simulink model "regs_12B_with_contracts_All_SLDV"  (R2017b)
settings: Solver=FixedStepDiscrete  StartTime=0.0  StopTime=10.0  FixedStep=0.200000  RelTol=1e-3  EnableMultiTasking=on
model workspace (MAT data in the model file):
  ContractValidatorBlocksMap = containers.Map
  ContractValidatorBlocksMap.serialization.keys = {'regs_12B_with_contracts/regs_12B_RegulatorSpec/validator', 'regs_12B_with_contracts_All/regs_12B_RegulatorSpec/validator'}
  ContractValidatorBlocksMap.serialization.values{1}.block = 'regs_12B_with_contracts/regs_12B_RegulatorSpec/validator'
  ContractValidatorBlocksMap.serialization.values{1}.assumePorts = 0
  ContractValidatorBlocksMap.serialization.values{1}.guaranteePorts = 10
  ContractValidatorBlocksMap.serialization.values{1}.modeBlocksPorts = 0
  ContractValidatorBlocksMap.serialization.values{1}.portHandles.Inport = [5912.00012207 5913.00012207 5914.00012207 5915.00012207 5916.00012207 5917.00012207 5918.00012207 5919.00012207 5920.00012207 5921.00012207]
  ContractValidatorBlocksMap.serialization.values{1}.portHandles.Outport = 5922.00012207
  ContractValidatorBlocksMap.serialization.values{1}.portHandles.Enable = []
  ContractValidatorBlocksMap.serialization.values{1}.portHandles.Trigger = []
  ContractValidatorBlocksMap.serialization.values{1}.portHandles.State = []
  ContractValidatorBlocksMap.serialization.values{1}.portHandles.LConn = []
  ContractValidatorBlocksMap.serialization.values{1}.portHandles.RConn = []
  ContractValidatorBlocksMap.serialization.values{1}.portHandles.Ifaction = []
  ContractValidatorBlocksMap.serialization.values{1}.portHandles.Reset = []
  ContractValidatorBlocksMap.serialization.values{1}.portConnectivity(1).Type = '1'
  ContractValidatorBlocksMap.serialization.values{1}.portConnectivity(1).Position = [138210 -150]
  ContractValidatorBlocksMap.serialization.values{1}.portConnectivity(1).SrcBlock = 5604.00012207
  ContractValidatorBlocksMap.serialization.values{1}.portConnectivity(1).SrcPort = 0
  ContractValidatorBlocksMap.serialization.values{1}.portConnectivity(1).DstBlock = []
  ContractValidatorBlocksMap.serialization.values{1}.portConnectivity(1).DstPort = []
  ContractValidatorBlocksMap.serialization.values{1}.portConnectivity(2).Type = '2'
  ContractValidatorBlocksMap.serialization.values{1}.portConnectivity(2).Position = [138210 -100]
  ContractValidatorBlocksMap.serialization.values{1}.portConnectivity(2).SrcBlock = 5608.00012207
  ContractValidatorBlocksMap.serialization.values{1}.portConnectivity(2).SrcPort = 0
  ContractValidatorBlocksMap.serialization.values{1}.portConnectivity(2).DstBlock = []
  ContractValidatorBlocksMap.serialization.values{1}.portConnectivity(2).DstPort = []
  ContractValidatorBlocksMap.serialization.values{1}.portConnectivity(3).Type = '3'
  ContractValidatorBlocksMap.serialization.values{1}.portConnectivity(3).Position = [138210 -50]
  ContractValidatorBlocksMap.serialization.values{1}.portConnectivity(3).SrcBlock = 5612.00012207
  ContractValidatorBlocksMap.serialization.values{1}.portConnectivity(3).SrcPort = 0
  ContractValidatorBlocksMap.serialization.values{1}.portConnectivity(3).DstBlock = []
  ContractValidatorBlocksMap.serialization.values{1}.portConnectivity(3).DstPort = []
  ContractValidatorBlocksMap.serialization.values{1}.portConnectivity(4).Type = '4'
  ContractValidatorBlocksMap.serialization.values{1}.portConnectivity(4).Position = [138210 0]
  ContractValidatorBlocksMap.serialization.values{1}.portConnectivity(4).SrcBlock = 5616.00012207
  ContractValidatorBlocksMap.serialization.values{1}.portConnectivity(4).SrcPort = 0
  ContractValidatorBlocksMap.serialization.values{1}.portConnectivity(4).DstBlock = []
  ContractValidatorBlocksMap.serialization.values{1}.portConnectivity(4).DstPort = []
  ContractValidatorBlocksMap.serialization.values{1}.portConnectivity(5).Type = '5'
  ContractValidatorBlocksMap.serialization.values{1}.portConnectivity(5).Position = [138210 50]
  ContractValidatorBlocksMap.serialization.values{1}.portConnectivity(5).SrcBlock = 5620.00012207
  ContractValidatorBlocksMap.serialization.values{1}.portConnectivity(5).SrcPort = 0
  ContractValidatorBlocksMap.serialization.values{1}.portConnectivity(5).DstBlock = []
  ContractValidatorBlocksMap.serialization.values{1}.portConnectivity(5).DstPort = []
  ContractValidatorBlocksMap.serialization.values{1}.portConnectivity(6).Type = '6'
  ContractValidatorBlocksMap.serialization.values{1}.portConnectivity(6).Position = [138210 100]
  ContractValidatorBlocksMap.serialization.values{1}.portConnectivity(6).SrcBlock = 5624.00012207
  ContractValidatorBlocksMap.serialization.values{1}.portConnectivity(6).SrcPort = 0
  ContractValidatorBlocksMap.serialization.values{1}.portConnectivity(6).DstBlock = []
  ContractValidatorBlocksMap.serialization.values{1}.portConnectivity(6).DstPort = []
  ContractValidatorBlocksMap.serialization.values{1}.portConnectivity(7).Type = '7'
  ContractValidatorBlocksMap.serialization.values{1}.portConnectivity(7).Position = [138210 150]
  ContractValidatorBlocksMap.serialization.values{1}.portConnectivity(7).SrcBlock = 5628.00012207
  ContractValidatorBlocksMap.serialization.values{1}.portConnectivity(7).SrcPort = 0
  ContractValidatorBlocksMap.serialization.values{1}.portConnectivity(7).DstBlock = []
  ContractValidatorBlocksMap.serialization.values{1}.portConnectivity(7).DstPort = []
  ContractValidatorBlocksMap.serialization.values{1}.portConnectivity(8).Type = '8'
  ContractValidatorBlocksMap.serialization.values{1}.portConnectivity(8).Position = [138210 200]
  ContractValidatorBlocksMap.serialization.values{1}.portConnectivity(8).SrcBlock = 5632.00012207
  ContractValidatorBlocksMap.serialization.values{1}.portConnectivity(8).SrcPort = 0
  ContractValidatorBlocksMap.serialization.values{1}.portConnectivity(8).DstBlock = []
  ContractValidatorBlocksMap.serialization.values{1}.portConnectivity(8).DstPort = []
  ContractValidatorBlocksMap.serialization.values{1}.portConnectivity(9).Type = '9'
  ContractValidatorBlocksMap.serialization.values{1}.portConnectivity(9).Position = [138210 250]
  ContractValidatorBlocksMap.serialization.values{1}.portConnectivity(9).SrcBlock = 5636.00012207
  ContractValidatorBlocksMap.serialization.values{1}.portConnectivity(9).SrcPort = 0
  ContractValidatorBlocksMap.serialization.values{1}.portConnectivity(9).DstBlock = []
  ContractValidatorBlocksMap.serialization.values{1}.portConnectivity(9).DstPort = []
  ContractValidatorBlocksMap.serialization.values{1}.portConnectivity(10).Type = '10'
  ContractValidatorBlocksMap.serialization.values{1}.portConnectivity(10).Position = [138210 300]
  ContractValidatorBlocksMap.serialization.values{1}.portConnectivity(10).SrcBlock = 5640.00012207
  ContractValidatorBlocksMap.serialization.values{1}.portConnectivity(10).SrcPort = 0
  ContractValidatorBlocksMap.serialization.values{1}.portConnectivity(10).DstBlock = []
  ContractValidatorBlocksMap.serialization.values{1}.portConnectivity(10).DstPort = []
  ContractValidatorBlocksMap.serialization.values{1}.portConnectivity(11).Type = '1'
  ContractValidatorBlocksMap.serialization.values{1}.portConnectivity(11).Position = [138345 75]
  ContractValidatorBlocksMap.serialization.values{1}.portConnectivity(11).SrcBlock = []
  ContractValidatorBlocksMap.serialization.values{1}.portConnectivity(11).SrcPort = []
  ContractValidatorBlocksMap.serialization.values{1}.portConnectivity(11).DstBlock = 5703.00012207
  ContractValidatorBlocksMap.serialization.values{1}.portConnectivity(11).DstPort = 0
  ContractValidatorBlocksMap.serialization.values{2}.block = 'regs_12B_with_contracts_All/regs_12B_RegulatorSpec/validator'
  ContractValidatorBlocksMap.serialization.values{2}.assumePorts = 0
  ContractValidatorBlocksMap.serialization.values{2}.guaranteePorts = 10
  ContractValidatorBlocksMap.serialization.values{2}.modeBlocksPorts = 0
  ContractValidatorBlocksMap.serialization.values{2}.portHandles.Inport = [7124.00512695 7125.00512695 7126.00512695 7127.00512695 7128.00512695 7129.00512695 7130.00512695 7131.00512695 7132.00512695 7133.00512695]
  ContractValidatorBlocksMap.serialization.values{2}.portHandles.Outport = 7134.00512695
  ContractValidatorBlocksMap.serialization.values{2}.portHandles.Enable = []
  ContractValidatorBlocksMap.serialization.values{2}.portHandles.Trigger = []
  ContractValidatorBlocksMap.serialization.values{2}.portHandles.State = []
  ContractValidatorBlocksMap.serialization.values{2}.portHandles.LConn = []
  ContractValidatorBlocksMap.serialization.values{2}.portHandles.RConn = []
  ContractValidatorBlocksMap.serialization.values{2}.portHandles.Ifaction = []
  ContractValidatorBlocksMap.serialization.values{2}.portHandles.Reset = []
  ContractValidatorBlocksMap.serialization.values{2}.portConnectivity(1).Type = '1'
  ContractValidatorBlocksMap.serialization.values{2}.portConnectivity(1).Position = [138210 -150]
  ContractValidatorBlocksMap.serialization.values{2}.portConnectivity(1).SrcBlock = 6800.00512695
  ContractValidatorBlocksMap.serialization.values{2}.portConnectivity(1).SrcPort = 0
  ContractValidatorBlocksMap.serialization.values{2}.portConnectivity(1).DstBlock = []
  ContractValidatorBlocksMap.serialization.values{2}.portConnectivity(1).DstPort = []
  ContractValidatorBlocksMap.serialization.values{2}.portConnectivity(2).Type = '2'
  ContractValidatorBlocksMap.serialization.values{2}.portConnectivity(2).Position = [138210 -100]
  ContractValidatorBlocksMap.serialization.values{2}.portConnectivity(2).SrcBlock = 6808.00512695
  ContractValidatorBlocksMap.serialization.values{2}.portConnectivity(2).SrcPort = 0
  ContractValidatorBlocksMap.serialization.values{2}.portConnectivity(2).DstBlock = []
  ContractValidatorBlocksMap.serialization.values{2}.portConnectivity(2).DstPort = []
  ContractValidatorBlocksMap.serialization.values{2}.portConnectivity(3).Type = '3'
  ContractValidatorBlocksMap.serialization.values{2}.portConnectivity(3).Position = [138210 -50]
  ContractValidatorBlocksMap.serialization.values{2}.portConnectivity(3).SrcBlock = 6812.00512695
  ContractValidatorBlocksMap.serialization.values{2}.portConnectivity(3).SrcPort = 0
  ContractValidatorBlocksMap.serialization.values{2}.portConnectivity(3).DstBlock = []
  ContractValidatorBlocksMap.serialization.values{2}.portConnectivity(3).DstPort = []
  ContractValidatorBlocksMap.serialization.values{2}.portConnectivity(4).Type = '4'
  ContractValidatorBlocksMap.serialization.values{2}.portConnectivity(4).Position = [138210 0]
  ContractValidatorBlocksMap.serialization.values{2}.portConnectivity(4).SrcBlock = 6816.00512695
  ContractValidatorBlocksMap.serialization.values{2}.portConnectivity(4).SrcPort = 0
  ContractValidatorBlocksMap.serialization.values{2}.portConnectivity(4).DstBlock = []
  ContractValidatorBlocksMap.serialization.values{2}.portConnectivity(4).DstPort = []
  ContractValidatorBlocksMap.serialization.values{2}.portConnectivity(5).Type = '5'
  ContractValidatorBlocksMap.serialization.values{2}.portConnectivity(5).Position = [138210 50]
  ContractValidatorBlocksMap.serialization.values{2}.portConnectivity(5).SrcBlock = 6820.00512695
  ContractValidatorBlocksMap.serialization.values{2}.portConnectivity(5).SrcPort = 0
  ContractValidatorBlocksMap.serialization.values{2}.portConnectivity(5).DstBlock = []
  ContractValidatorBlocksMap.serialization.values{2}.portConnectivity(5).DstPort = []
  ContractValidatorBlocksMap.serialization.values{2}.portConnectivity(6).Type = '6'
  ContractValidatorBlocksMap.serialization.values{2}.portConnectivity(6).Position = [138210 100]
  ContractValidatorBlocksMap.serialization.values{2}.portConnectivity(6).SrcBlock = 6824.00512695
  ContractValidatorBlocksMap.serialization.values{2}.portConnectivity(6).SrcPort = 0
  ContractValidatorBlocksMap.serialization.values{2}.portConnectivity(6).DstBlock = []
  ContractValidatorBlocksMap.serialization.values{2}.portConnectivity(6).DstPort = []
  ContractValidatorBlocksMap.serialization.values{2}.portConnectivity(7).Type = '7'
  ContractValidatorBlocksMap.serialization.values{2}.portConnectivity(7).Position = [138210 150]
  ContractValidatorBlocksMap.serialization.values{2}.portConnectivity(7).SrcBlock = 6828.00512695
  ContractValidatorBlocksMap.serialization.values{2}.portConnectivity(7).SrcPort = 0
  ContractValidatorBlocksMap.serialization.values{2}.portConnectivity(7).DstBlock = []
  ContractValidatorBlocksMap.serialization.values{2}.portConnectivity(7).DstPort = []
  ContractValidatorBlocksMap.serialization.values{2}.portConnectivity(8).Type = '8'
  ContractValidatorBlocksMap.serialization.values{2}.portConnectivity(8).Position = [138210 200]
  ContractValidatorBlocksMap.serialization.values{2}.portConnectivity(8).SrcBlock = 6832.00512695
  ContractValidatorBlocksMap.serialization.values{2}.portConnectivity(8).SrcPort = 0
  ContractValidatorBlocksMap.serialization.values{2}.portConnectivity(8).DstBlock = []
  ContractValidatorBlocksMap.serialization.values{2}.portConnectivity(8).DstPort = []
  ContractValidatorBlocksMap.serialization.values{2}.portConnectivity(9).Type = '9'
  ContractValidatorBlocksMap.serialization.values{2}.portConnectivity(9).Position = [138210 250]
  ContractValidatorBlocksMap.serialization.values{2}.portConnectivity(9).SrcBlock = 6836.00512695
  ContractValidatorBlocksMap.serialization.values{2}.portConnectivity(9).SrcPort = 0
  ContractValidatorBlocksMap.serialization.values{2}.portConnectivity(9).DstBlock = []
  ContractValidatorBlocksMap.serialization.values{2}.portConnectivity(9).DstPort = []
  ContractValidatorBlocksMap.serialization.values{2}.portConnectivity(10).Type = '10'
  ContractValidatorBlocksMap.serialization.values{2}.portConnectivity(10).Position = [138210 300]
  ContractValidatorBlocksMap.serialization.values{2}.portConnectivity(10).SrcBlock = 6804.00512695
  ContractValidatorBlocksMap.serialization.values{2}.portConnectivity(10).SrcPort = 0
  ContractValidatorBlocksMap.serialization.values{2}.portConnectivity(10).DstBlock = []
  ContractValidatorBlocksMap.serialization.values{2}.portConnectivity(10).DstPort = []
  ContractValidatorBlocksMap.serialization.values{2}.portConnectivity(11).Type = '1'
  ContractValidatorBlocksMap.serialization.values{2}.portConnectivity(11).Position = [138345 75]
  ContractValidatorBlocksMap.serialization.values{2}.portConnectivity(11).SrcBlock = []
  ContractValidatorBlocksMap.serialization.values{2}.portConnectivity(11).SrcPort = []
  ContractValidatorBlocksMap.serialization.values{2}.portConnectivity(11).DstBlock = 6915.00512695
  ContractValidatorBlocksMap.serialization.values{2}.portConnectivity(11).DstPort = 0
  ContractValidatorBlocksMap.serialization.uniformity = 0
  ContractValidatorBlocksMap.serialization.keyType = 'char'
  ContractValidatorBlocksMap.serialization.valueType = 'any'
undefined symbols (not defined in the file): dt, transition_v, transition_y
libraries: sldvlib x10, simulink x2
settings Model: Creator=elliocm  LastModifiedBy=hbourbou
settings DataIOCC: LimitDataPoints=on  SaveFormat=Array  SignalLoggingSaveFormat=ModelDataLogs
settings OptimizationCC: ExpressionDepthLimit=2147483647  LifeSpan=inf
settings DebuggingCC: UnderspecifiedInitializationDetection=Classic  MergeDetectMultiDrivingBlocksExec=none  SolverPrmCheckMsg=warning  FcnCallInpInsideContextMsg=warning  StateNameClashWarn=warning  SFUnexpectedBacktrackingDiag=warning  SFNoUnconditionalDefaultTransitionDiag=warning  SFExecutionAtInitializationDiag=none
settings HardwareCC: ProdBitPerPointer=32  ProdBitPerSizeT=32  ProdBitPerPtrDiffT=32  ProdLargestAtomicFloat=None  ProdIntDivRoundTo=Undefined  ProdEndianess=Unspecified  ProdWordSize=32  ProdHWDeviceType=32-bit Generic
settings ModelReferenceCC: PropagateSignalLabelsOutOfModel=off
settings CodeAppCC: StateflowObjectComments=on
settings GRTTargetCC: TargetLangStandard=C89/C90 (ANSI)  GeneratePreprocessorConditionals=Disable all  CombineOutputUpdateFcns=off  GRTInterface=on
settings ConfigComp: CovMetricSettings=dw  CovHtmlReporting=on  CovSaveCumulativeToWorkspaceVar=on  CovSaveSingleToWorkspaceVar=on  CovExternalEMLEnable=off  DVMode=PropertyProving  DVMaxProcessTime=7200  DVTestSuiteOptimization=CombinedObjectives (Nonlinear Extended)  DVDetectOutOfBounds=on

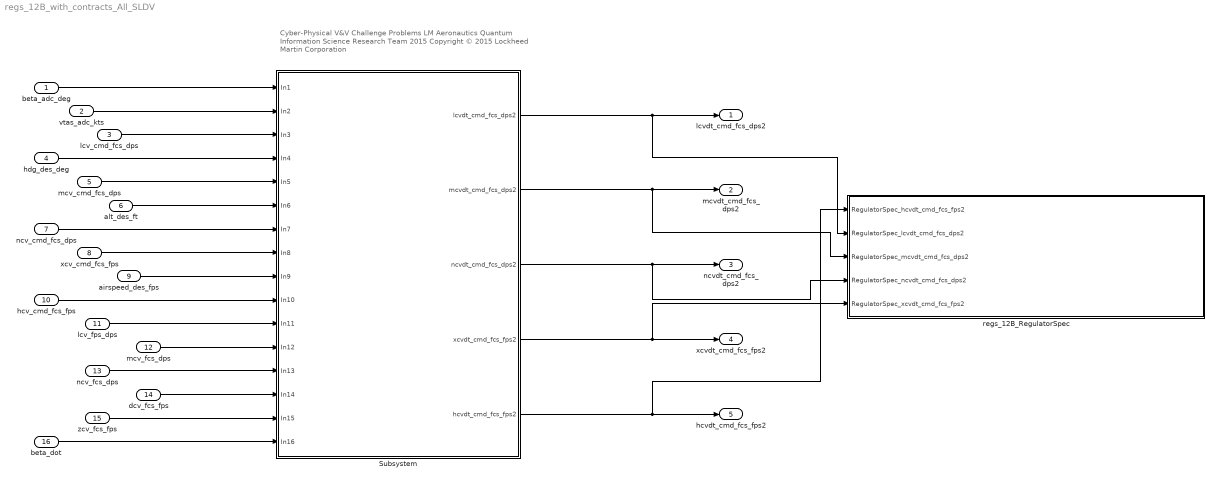
== system regs_12B_with_contracts_All_SLDV ==
  note: Cyber-Physical V&V Challenge Problems
      | LM Aeronautics Quantum Information Science Research Team 2015
      | Copyright © 2015 Lockheed Martin Corporation
  beta_adc_deg : Inport  OutDataTypeStr=double
  vtas_adc_kts : Inport  Port=2  OutDataTypeStr=double
  "lcv_cmd_fcs_dps " : Inport  Port=3  OutDataTypeStr=double
  hdg_des_deg : Inport  Port=4  OutDataTypeStr=double
  mcv_cmd_fcs_dps : Inport  Port=5  OutDataTypeStr=double
  alt_des_ft : Inport  Port=6  OutDataTypeStr=double
  ncv_cmd_fcs_dps : Inport  Port=7  OutDataTypeStr=double
  xcv_cmd_fcs_fps : Inport  Port=8  OutDataTypeStr=double
  airspeed_des_fps : Inport  Port=9  OutDataTypeStr=double
  hcv_cmd_fcs_fps : Inport  Port=10  OutDataTypeStr=double
  lcv_fps_dps : Inport  Port=11  OutDataTypeStr=double
  mcv_fcs_dps : Inport  Port=12  OutDataTypeStr=double
  ncv_fcs_dps : Inport  Port=13  OutDataTypeStr=double
  dcv_fcs_fps : Inport  Port=14  OutDataTypeStr=double
  zcv_fcs_fps : Inport  Port=15  OutDataTypeStr=double
  beta_dot : Inport  Port=16  OutDataTypeStr=double
  Subsystem : Subsystem
  regs_12B_RegulatorSpec : Subsystem  TreatAsAtomicUnit=on  SimViewingDevice=on  mask(VerificationSubsystem){}
      mask Display: image(imread('sldvicon_versubsys.png','BackGroundColor',[1 1 1]),'center');
  lcvdt_cmd_fcs_dps2 : Outport  VectorParamsAs1DForOutWhenUnconnected=off
  mcvdt_cmd_fcs_dps2 : Outport  Port=2  VectorParamsAs1DForOutWhenUnconnected=off
  ncvdt_cmd_fcs_dps2 : Outport  Port=3  VectorParamsAs1DForOutWhenUnconnected=off
  xcvdt_cmd_fcs_fps2 : Outport  Port=4  VectorParamsAs1DForOutWhenUnconnected=off
  hcvdt_cmd_fcs_fps2 : Outport  Port=5  VectorParamsAs1DForOutWhenUnconnected=off
  wires:
  beta_adc_deg/1 -> Subsystem/1(In1)
  vtas_adc_kts/1 -> Subsystem/2(In2)
  "lcv_cmd_fcs_dps "/1 -> Subsystem/3(In3)
  hdg_des_deg/1 -> Subsystem/4(In4)
  mcv_cmd_fcs_dps/1 -> Subsystem/5(In5)
  alt_des_ft/1 -> Subsystem/6(In6)
  ncv_cmd_fcs_dps/1 -> Subsystem/7(In7)
  xcv_cmd_fcs_fps/1 -> Subsystem/8(In8)
  airspeed_des_fps/1 -> Subsystem/9(In9)
  hcv_cmd_fcs_fps/1 -> Subsystem/10(In10)
  lcv_fps_dps/1 -> Subsystem/11(In11)
  mcv_fcs_dps/1 -> Subsystem/12(In12)
  ncv_fcs_dps/1 -> Subsystem/13(In13)
  dcv_fcs_fps/1 -> Subsystem/14(In14)
  zcv_fcs_fps/1 -> Subsystem/15(In15)
  beta_dot/1 -> Subsystem/16(In16)
  Subsystem/1(lcvdt_cmd_fcs_dps2) -> lcvdt_cmd_fcs_dps2/1, regs_12B_RegulatorSpec/2(RegulatorSpec_lcvdt_cmd_fcs_dps2)
  Subsystem/2(mcvdt_cmd_fcs_dps2) -> mcvdt_cmd_fcs_dps2/1, regs_12B_RegulatorSpec/3(RegulatorSpec_mcvdt_cmd_fcs_dps2)
  Subsystem/3(ncvdt_cmd_fcs_dps2) -> ncvdt_cmd_fcs_dps2/1, regs_12B_RegulatorSpec/4(RegulatorSpec_ncvdt_cmd_fcs_dps2)
  Subsystem/4(xcvdt_cmd_fcs_fps2) -> xcvdt_cmd_fcs_fps2/1, regs_12B_RegulatorSpec/5(RegulatorSpec_xcvdt_cmd_fcs_fps2)
  Subsystem/5(hcvdt_cmd_fcs_fps2) -> hcvdt_cmd_fcs_fps2/1, regs_12B_RegulatorSpec/1(RegulatorSpec_hcvdt_cmd_fcs_fps2)

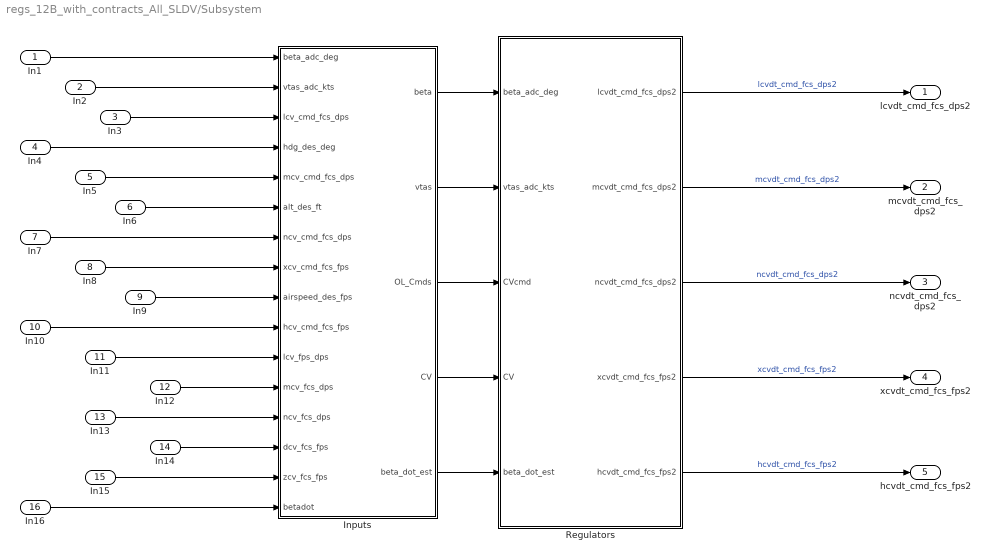
== system regs_12B_with_contracts_All_SLDV/Subsystem ==
  In1 : Inport
  In2 : Inport  Port=2
  In3 : Inport  Port=3
  In4 : Inport  Port=4
  In5 : Inport  Port=5
  In6 : Inport  Port=6
  In7 : Inport  Port=7
  In8 : Inport  Port=8
  In9 : Inport  Port=9
  In10 : Inport  Port=10
  In11 : Inport  Port=11
  In12 : Inport  Port=12
  In13 : Inport  Port=13
  In14 : Inport  Port=14
  In15 : Inport  Port=15
  In16 : Inport  Port=16
  Inputs : Subsystem
  Regulators : Subsystem
  lcvdt_cmd_fcs_dps2 : Outport
  mcvdt_cmd_fcs_dps2 : Outport  Port=2
  ncvdt_cmd_fcs_dps2 : Outport  Port=3
  xcvdt_cmd_fcs_fps2 : Outport  Port=4
  hcvdt_cmd_fcs_fps2 : Outport  Port=5
  wires:
  In12/1 -> Inputs/12(mcv_fcs_dps)
  In6/1 -> Inputs/6(alt_des_ft)
  Regulators/2(mcvdt_cmd_fcs_dps2) -> mcvdt_cmd_fcs_dps2/1  "mcvdt_cmd_fcs_dps2"
  Inputs/4(CV) -> Regulators/4(CV)
  Regulators/3(ncvdt_cmd_fcs_dps2) -> ncvdt_cmd_fcs_dps2/1  "ncvdt_cmd_fcs_dps2"
  In11/1 -> Inputs/11(lcv_fps_dps)
  In14/1 -> Inputs/14(dcv_fcs_fps)
  In3/1 -> Inputs/3("lcv_cmd_fcs_dps ")
  Inputs/5(beta_dot_est) -> Regulators/5(beta_dot_est)
  Regulators/5(hcvdt_cmd_fcs_fps2) -> hcvdt_cmd_fcs_fps2/1  "hcvdt_cmd_fcs_fps2"
  Inputs/3(OL_Cmds) -> Regulators/3(CVcmd)
  In2/1 -> Inputs/2(vtas_adc_kts)
  In4/1 -> Inputs/4(hdg_des_deg)
  In10/1 -> Inputs/10(hcv_cmd_fcs_fps)
  In5/1 -> Inputs/5(mcv_cmd_fcs_dps)
  In13/1 -> Inputs/13(ncv_fcs_dps)
  Regulators/1(lcvdt_cmd_fcs_dps2) -> lcvdt_cmd_fcs_dps2/1  "lcvdt_cmd_fcs_dps2"
  In8/1 -> Inputs/8(xcv_cmd_fcs_fps)
  Inputs/1(beta) -> Regulators/1(beta_adc_deg)
  In7/1 -> Inputs/7(ncv_cmd_fcs_dps)
  In16/1 -> Inputs/16(betadot)
  In1/1 -> Inputs/1(beta_adc_deg)
  In9/1 -> Inputs/9(airspeed_des_fps)
  In15/1 -> Inputs/15(zcv_fcs_fps)
  Inputs/2(vtas) -> Regulators/2(vtas_adc_kts)
  Regulators/4(xcvdt_cmd_fcs_fps2) -> xcvdt_cmd_fcs_fps2/1  "xcvdt_cmd_fcs_fps2"

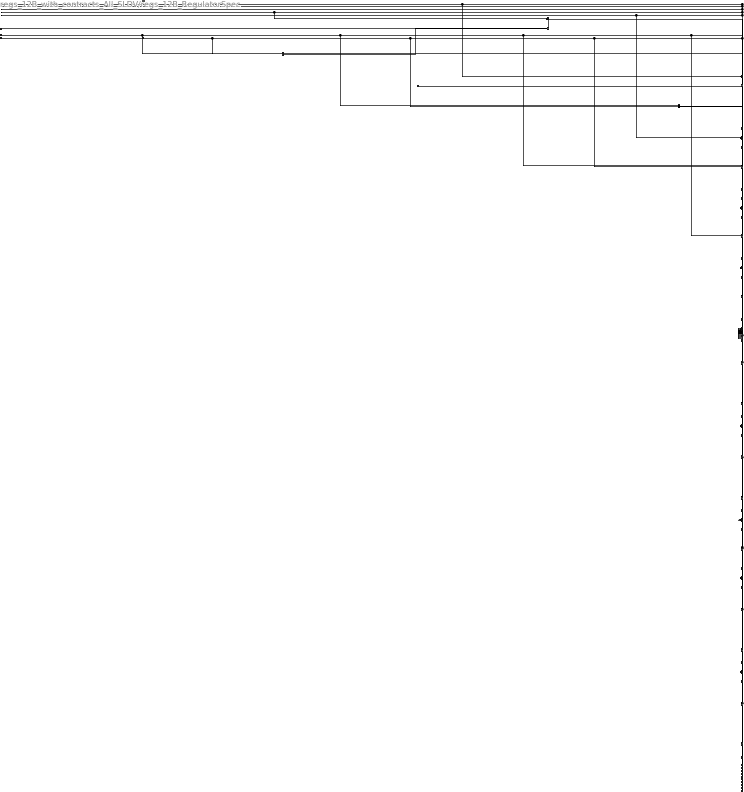
== system regs_12B_with_contracts_All_SLDV/regs_12B_RegulatorSpec ==
  RegulatorSpec_hcvdt_cmd_fcs_fps2 : Inport  OutDataTypeStr=double
  RegulatorSpec_lcvdt_cmd_fcs_dps2 : Inport  Port=2  OutDataTypeStr=double
  RegulatorSpec_mcvdt_cmd_fcs_dps2 : Inport  Port=3  OutDataTypeStr=double
  RegulatorSpec_ncvdt_cmd_fcs_dps2 : Inport  Port=4  OutDataTypeStr=double
  RegulatorSpec_xcvdt_cmd_fcs_fps2 : Inport  Port=5  OutDataTypeStr=double
  Arrow_xxRegulatorSpec_1_ni_7 : Delay  DelayLength=1  InitialCondition=1
  Assertion{1..10} (10 alike) : sldvlib/Objectives and Constraints/Proof Objective  enabled=on  customAVTBlockType=Proof Objective  intervals=true  dispValues=on  outEnabled=off  enableStopSim=off
      settings: AttributesFormatString=%<intervals>  SourceProductName=Simulink  SourceProductBaseCode=SL
  PRE_xxRegulatorSpec_{4,8,12,15,19,23,27,31,35,39} (10 alike) : Delay  DelayLength=1  InitialCondition=0
  REG001 : Subsystem
  REG0010 : Subsystem
  REG002 : Subsystem
  REG003 : Subsystem
  REG004 : Subsystem
  REG005 : Subsystem
  REG006 : Subsystem
  REG007 : Subsystem
  REG008 : Subsystem
  REG009 : Subsystem
  branch_10_IF : Switch  Criteria=u2 ~= 0
  branch_11_IF : Switch  Criteria=u2 ~= 0
  branch_12_IF : Switch  Criteria=u2 ~= 0
  branch_13_IF : Switch  Criteria=u2 ~= 0
  branch_14_IF : Switch  Criteria=u2 ~= 0
  branch_15_IF : Switch  Criteria=u2 ~= 0
  branch_16_IF : Switch  Criteria=u2 ~= 0
  branch_17_IF : Switch  Criteria=u2 ~= 0
  branch_18_IF : Switch  Criteria=u2 ~= 0
  branch_19_IF : Switch  Criteria=u2 ~= 0
  branch_6_IF : Switch  Criteria=u2 ~= 0
  branch_7_IF : Switch  Criteria=u2 ~= 0
  branch_8_IF : Switch  Criteria=u2 ~= 0
  branch_9_IF : Switch  Criteria=u2 ~= 0
  spec126_operator : RelationalOperator  Operator=<=  OutDataTypeStr=boolean  RndMeth=Simplest
  spec126_rhs_2 : Constant  Value=100  OutDataTypeStr=int32
  spec144_operator : RelationalOperator  Operator=<=  OutDataTypeStr=boolean  RndMeth=Simplest
  spec144_rhs_2 : Constant  Value=100  OutDataTypeStr=int32
  spec160_operator : RelationalOperator  Operator=<=  OutDataTypeStr=boolean  RndMeth=Simplest
  spec160_rhs_2 : Constant  Value=100  OutDataTypeStr=int32
  spec178_operator : RelationalOperator  Operator=<=  OutDataTypeStr=boolean  RndMeth=Simplest
  spec178_rhs_2 : Constant  Value=100  OutDataTypeStr=int32
  spec196_operator : RelationalOperator  Operator=<=  OutDataTypeStr=boolean  RndMeth=Simplest
  spec196_rhs_2 : Constant  Value=100  OutDataTypeStr=int32
  spec211_operator : RelationalOperator  Operator=<=  OutDataTypeStr=boolean  RndMeth=Simplest
  spec211_rhs_2 : Constant  Value=50.0  OutDataTypeStr=double
  spec226_operator : RelationalOperator  Operator=<=  OutDataTypeStr=boolean  RndMeth=Simplest
  spec226_rhs_2 : Constant  Value=50.0  OutDataTypeStr=double
  spec241_operator : RelationalOperator  Operator=<=  OutDataTypeStr=boolean  RndMeth=Simplest
  spec241_rhs_2 : Constant  Value=50.0  OutDataTypeStr=double
  spec256_operator : RelationalOperator  Operator=<=  OutDataTypeStr=boolean  RndMeth=Simplest
  spec256_rhs_2 : Constant  Value=32.0  OutDataTypeStr=double
  spec271_operator : RelationalOperator  Operator=<=  OutDataTypeStr=boolean  RndMeth=Simplest
  spec271_rhs_2 : Constant  Value=32.0  OutDataTypeStr=double
  xxRegulatorSpec_11_operator : RelationalOperator  Operator=>  OutDataTypeStr=boolean  RndMeth=Simplest
  xxRegulatorSpec_11_rhs_2 : Constant  Value=50.0  OutDataTypeStr=double
  xxRegulatorSpec_13_operator : Sum  OutDataTypeStr=int32
  xxRegulatorSpec_13_rhs_2 : Constant  OutDataTypeStr=int32
  xxRegulatorSpec_14_operator : RelationalOperator  Operator=>  OutDataTypeStr=boolean  RndMeth=Simplest
  xxRegulatorSpec_14_rhs_2 : Constant  Value=32.0  OutDataTypeStr=double
  xxRegulatorSpec_16_operator : Sum  OutDataTypeStr=int32
  xxRegulatorSpec_16_rhs_2 : Constant  OutDataTypeStr=int32
  xxRegulatorSpec_18_operator : RelationalOperator  Operator=>  OutDataTypeStr=boolean  RndMeth=Simplest
  xxRegulatorSpec_18_rhs_2 : Constant  Value=32.0  OutDataTypeStr=double
  xxRegulatorSpec_1_ni_7_init : Constant  Value=0  OutDataTypeStr=boolean
  xxRegulatorSpec_20_operator : Sum  OutDataTypeStr=int32
  xxRegulatorSpec_20_rhs_2 : Constant  OutDataTypeStr=int32
  xxRegulatorSpec_22_rhs : Constant  Value=0.0  OutDataTypeStr=double
  xxRegulatorSpec_24_operator : Sum  Inputs=+-  OutDataTypeStr=double
  xxRegulatorSpec_25_operator : Product  OutDataTypeStr=double
  xxRegulatorSpec_25_rhs_2 : Constant  Value=100.0  OutDataTypeStr=double
  xxRegulatorSpec_28_operator : Sum  Inputs=+-  OutDataTypeStr=double
  xxRegulatorSpec_29_operator : Product  OutDataTypeStr=double
  xxRegulatorSpec_29_rhs_2 : Constant  Value=100.0  OutDataTypeStr=double
  xxRegulatorSpec_2_rhs : Constant  Value=0  OutDataTypeStr=Inherit: Inherit via back propagation
  xxRegulatorSpec_32_operator : Sum  Inputs=+-  OutDataTypeStr=double
  xxRegulatorSpec_33_operator : Product  OutDataTypeStr=double
  xxRegulatorSpec_33_rhs_2 : Constant  Value=100.0  OutDataTypeStr=double
  xxRegulatorSpec_36_operator : Sum  Inputs=+-  OutDataTypeStr=double
  xxRegulatorSpec_37_operator : Product  OutDataTypeStr=double
  xxRegulatorSpec_37_rhs_2 : Constant  Value=100.0  OutDataTypeStr=double
  xxRegulatorSpec_3_operator : RelationalOperator  Operator=>  OutDataTypeStr=boolean  RndMeth=Simplest
  xxRegulatorSpec_3_rhs_2 : Constant  Value=50.0  OutDataTypeStr=double
  xxRegulatorSpec_40_operator : Sum  Inputs=+-  OutDataTypeStr=double
  xxRegulatorSpec_41_operator : Product  OutDataTypeStr=double
  xxRegulatorSpec_41_rhs_2 : Constant  Value=100.0  OutDataTypeStr=double
  xxRegulatorSpec_5_operator : Sum  OutDataTypeStr=int32
  xxRegulatorSpec_5_rhs_2 : Constant  OutDataTypeStr=int32
  xxRegulatorSpec_7_operator : RelationalOperator  Operator=>  OutDataTypeStr=boolean  RndMeth=Simplest
  xxRegulatorSpec_7_rhs_2 : Constant  Value=50.0  OutDataTypeStr=double
  xxRegulatorSpec_9_operator : Sum  OutDataTypeStr=int32
  xxRegulatorSpec_9_rhs_2 : Constant  OutDataTypeStr=int32
  wires:
  xxRegulatorSpec_9_rhs_2/1 -> xxRegulatorSpec_9_operator/2
  PRE_xxRegulatorSpec_8/1 -> xxRegulatorSpec_9_operator/1
  xxRegulatorSpec_7_rhs_2/1 -> xxRegulatorSpec_7_operator/2
  xxRegulatorSpec_5_rhs_2/1 -> xxRegulatorSpec_5_operator/2
  PRE_xxRegulatorSpec_4/1 -> xxRegulatorSpec_5_operator/1
  xxRegulatorSpec_41_rhs_2/1 -> xxRegulatorSpec_41_operator/2
  xxRegulatorSpec_40_operator/1 -> xxRegulatorSpec_41_operator/1
  PRE_xxRegulatorSpec_39/1 -> xxRegulatorSpec_40_operator/2
  xxRegulatorSpec_3_rhs_2/1 -> xxRegulatorSpec_3_operator/2
  xxRegulatorSpec_37_rhs_2/1 -> xxRegulatorSpec_37_operator/2
  xxRegulatorSpec_36_operator/1 -> xxRegulatorSpec_37_operator/1
  PRE_xxRegulatorSpec_35/1 -> xxRegulatorSpec_36_operator/2
  xxRegulatorSpec_33_rhs_2/1 -> xxRegulatorSpec_33_operator/2
  xxRegulatorSpec_32_operator/1 -> xxRegulatorSpec_33_operator/1
  PRE_xxRegulatorSpec_31/1 -> xxRegulatorSpec_32_operator/2
  xxRegulatorSpec_29_rhs_2/1 -> xxRegulatorSpec_29_operator/2
  xxRegulatorSpec_28_operator/1 -> xxRegulatorSpec_29_operator/1
  PRE_xxRegulatorSpec_27/1 -> xxRegulatorSpec_28_operator/2
  xxRegulatorSpec_25_rhs_2/1 -> xxRegulatorSpec_25_operator/2
  xxRegulatorSpec_24_operator/1 -> xxRegulatorSpec_25_operator/1
  PRE_xxRegulatorSpec_23/1 -> xxRegulatorSpec_24_operator/2
  xxRegulatorSpec_20_rhs_2/1 -> xxRegulatorSpec_20_operator/2
  PRE_xxRegulatorSpec_19/1 -> xxRegulatorSpec_20_operator/1
  xxRegulatorSpec_18_rhs_2/1 -> xxRegulatorSpec_18_operator/2
  xxRegulatorSpec_16_rhs_2/1 -> xxRegulatorSpec_16_operator/2
  PRE_xxRegulatorSpec_15/1 -> xxRegulatorSpec_16_operator/1
  xxRegulatorSpec_14_rhs_2/1 -> xxRegulatorSpec_14_operator/2
  xxRegulatorSpec_13_rhs_2/1 -> xxRegulatorSpec_13_operator/2
  PRE_xxRegulatorSpec_12/1 -> xxRegulatorSpec_13_operator/1
  xxRegulatorSpec_11_rhs_2/1 -> xxRegulatorSpec_11_operator/2
  spec271_rhs_2/1 -> spec271_operator/2
  branch_7_IF/1 -> spec271_operator/1
  spec256_rhs_2/1 -> spec256_operator/2
  branch_8_IF/1 -> spec256_operator/1
  spec241_rhs_2/1 -> spec241_operator/2
  branch_6_IF/1 -> spec241_operator/1
  spec226_rhs_2/1 -> spec226_operator/2
  branch_9_IF/1 -> spec226_operator/1
  spec211_rhs_2/1 -> spec211_operator/2
  branch_10_IF/1 -> spec211_operator/1
  spec196_rhs_2/1 -> spec196_operator/2
  spec178_rhs_2/1 -> spec178_operator/2
  spec160_rhs_2/1 -> spec160_operator/2
  spec144_rhs_2/1 -> spec144_operator/2
  spec126_rhs_2/1 -> spec126_operator/2
  spec271_operator/1 -> REG0010/1(In1)
  spec256_operator/1 -> REG009/1(In1)
  spec241_operator/1 -> REG008/1(In1)
  spec226_operator/1 -> REG007/1(In1)
  spec211_operator/1 -> REG006/1(In1)
  spec196_operator/1 -> REG005/1(In1)
  spec178_operator/1 -> REG004/1(In1)
  spec160_operator/1 -> REG003/1(In1)
  spec144_operator/1 -> REG002/1(In1)
  spec126_operator/1 -> REG001/1(In1)
  xxRegulatorSpec_13_operator/1 -> [a_e_count_yaw_output_exceeding_50]
  xxRegulatorSpec_29_operator/1 -> branch_9_IF/3
  xxRegulatorSpec_37_operator/1 -> branch_8_IF/3
  xxRegulatorSpec_41_operator/1 -> branch_7_IF/3
  xxRegulatorSpec_33_operator/1 -> branch_6_IF/3
  xxRegulatorSpec_3_operator/1 -> branch_19_IF/2
  xxRegulatorSpec_5_operator/1 -> branch_19_IF/1
  branch_19_IF/1 -> branch_18_IF/3
  xxRegulatorSpec_7_operator/1 -> branch_17_IF/2
  xxRegulatorSpec_9_operator/1 -> branch_17_IF/1
  branch_17_IF/1 -> branch_16_IF/3
  xxRegulatorSpec_11_operator/1 -> branch_15_IF/2
  xxRegulatorSpec_14_operator/1 -> branch_14_IF/2
  xxRegulatorSpec_16_operator/1 -> branch_14_IF/1
  branch_14_IF/1 -> branch_13_IF/3
  xxRegulatorSpec_18_operator/1 -> branch_12_IF/2
  xxRegulatorSpec_20_operator/1 -> branch_12_IF/1
  branch_12_IF/1 -> branch_11_IF/3
  xxRegulatorSpec_25_operator/1 -> branch_10_IF/3
  xxRegulatorSpec_1_ni_7_init/1 -> Arrow_xxRegulatorSpec_1_ni_7/1
  RegulatorSpec_lcvdt_cmd_fcs_dps2/1 -> xxRegulatorSpec_3_operator/1, PRE_xxRegulatorSpec_23/1, xxRegulatorSpec_24_operator/1
  RegulatorSpec_mcvdt_cmd_fcs_dps2/1 -> xxRegulatorSpec_7_operator/1, PRE_xxRegulatorSpec_27/1, xxRegulatorSpec_28_operator/1
  branch_18_IF/1 -> spec126_operator/1, PRE_xxRegulatorSpec_4/1
  branch_16_IF/1 -> spec144_operator/1, PRE_xxRegulatorSpec_8/1
  branch_15_IF/1 -> spec160_operator/1, PRE_xxRegulatorSpec_12/1
  RegulatorSpec_ncvdt_cmd_fcs_dps2/1 -> xxRegulatorSpec_11_operator/1, PRE_xxRegulatorSpec_31/1, xxRegulatorSpec_32_operator/1
  branch_13_IF/1 -> spec178_operator/1, PRE_xxRegulatorSpec_15/1
  RegulatorSpec_xcvdt_cmd_fcs_fps2/1 -> xxRegulatorSpec_14_operator/1, PRE_xxRegulatorSpec_35/1, xxRegulatorSpec_36_operator/1
  branch_11_IF/1 -> spec196_operator/1, PRE_xxRegulatorSpec_19/1
  xxRegulatorSpec_2_rhs/1 -> branch_15_IF/3, branch_15_IF/1, branch_19_IF/3, branch_18_IF/1, branch_17_IF/3, branch_16_IF/1, branch_14_IF/3, branch_13_IF/1, branch_12_IF/3, branch_11_IF/1
  RegulatorSpec_hcvdt_cmd_fcs_fps2/1 -> xxRegulatorSpec_18_operator/1, PRE_xxRegulatorSpec_39/1, xxRegulatorSpec_40_operator/1
  xxRegulatorSpec_22_rhs/1 -> branch_9_IF/1, branch_10_IF/1, branch_8_IF/1, branch_7_IF/1, branch_6_IF/1
  Arrow_xxRegulatorSpec_1_ni_7/1 -> branch_18_IF/2, branch_16_IF/2, branch_13_IF/2, branch_11_IF/2, branch_10_IF/2, branch_9_IF/2, branch_8_IF/2, branch_7_IF/2, branch_6_IF/2
  REG001/1(guarantee) -> Assertion1/1
  REG002/1(guarantee) -> Assertion2/1
  REG003/1(guarantee) -> Assertion3/1
  REG004/1(guarantee) -> Assertion4/1
  REG005/1(guarantee) -> Assertion5/1
  REG006/1(guarantee) -> Assertion6/1
  REG007/1(guarantee) -> Assertion7/1
  REG008/1(guarantee) -> Assertion8/1
  REG009/1(guarantee) -> Assertion9/1
  REG0010/1(guarantee) -> Assertion10/1

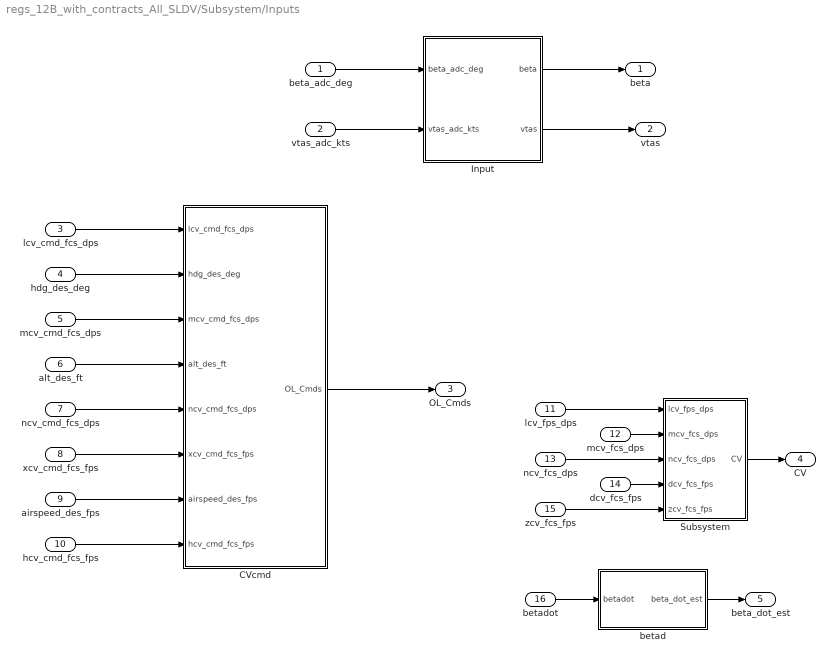
== system regs_12B_with_contracts_All_SLDV/Subsystem/Inputs ==
  beta_adc_deg : Inport
  vtas_adc_kts : Inport  Port=2
  "lcv_cmd_fcs_dps " : Inport  Port=3
  hdg_des_deg : Inport  Port=4
  mcv_cmd_fcs_dps : Inport  Port=5
  alt_des_ft : Inport  Port=6
  ncv_cmd_fcs_dps : Inport  Port=7
  xcv_cmd_fcs_fps : Inport  Port=8
  airspeed_des_fps : Inport  Port=9
  hcv_cmd_fcs_fps : Inport  Port=10
  lcv_fps_dps : Inport  Port=11
  mcv_fcs_dps : Inport  Port=12
  ncv_fcs_dps : Inport  Port=13
  dcv_fcs_fps : Inport  Port=14
  zcv_fcs_fps : Inport  Port=15
  betadot : Inport  Port=16
  CVcmd : Subsystem
  Input : Subsystem
  Subsystem : Subsystem
  betad : Subsystem
  beta : Outport  VectorParamsAs1DForOutWhenUnconnected=off
  vtas : Outport  Port=2  VectorParamsAs1DForOutWhenUnconnected=off
  OL_Cmds : Outport  Port=3  VectorParamsAs1DForOutWhenUnconnected=off
  CV : Outport  Port=4  VectorParamsAs1DForOutWhenUnconnected=off
  beta_dot_est : Outport  Port=5  VectorParamsAs1DForOutWhenUnconnected=off
  wires:
  Subsystem/1(CV) -> CV/1
  CVcmd/1(OL_Cmds) -> OL_Cmds/1
  beta_adc_deg/1 -> Input/1(beta_adc_deg)
  vtas_adc_kts/1 -> Input/2(vtas_adc_kts)
  "lcv_cmd_fcs_dps "/1 -> CVcmd/1("lcv_cmd_fcs_dps ")
  mcv_cmd_fcs_dps/1 -> CVcmd/3(mcv_cmd_fcs_dps)
  ncv_cmd_fcs_dps/1 -> CVcmd/5(ncv_cmd_fcs_dps)
  xcv_cmd_fcs_fps/1 -> CVcmd/6(xcv_cmd_fcs_fps)
  hcv_cmd_fcs_fps/1 -> CVcmd/8(hcv_cmd_fcs_fps)
  hdg_des_deg/1 -> CVcmd/2(hdg_des_deg)
  alt_des_ft/1 -> CVcmd/4(alt_des_ft)
  airspeed_des_fps/1 -> CVcmd/7(airspeed_des_fps)
  zcv_fcs_fps/1 -> Subsystem/5(zcv_fcs_fps)
  dcv_fcs_fps/1 -> Subsystem/4(dcv_fcs_fps)
  lcv_fps_dps/1 -> Subsystem/1(lcv_fps_dps)
  mcv_fcs_dps/1 -> Subsystem/2(mcv_fcs_dps)
  ncv_fcs_dps/1 -> Subsystem/3(ncv_fcs_dps)
  betadot/1 -> betad/1(betadot)
  betad/1(beta_dot_est) -> beta_dot_est/1
  Input/1(beta) -> beta/1
  Input/2(vtas) -> vtas/1

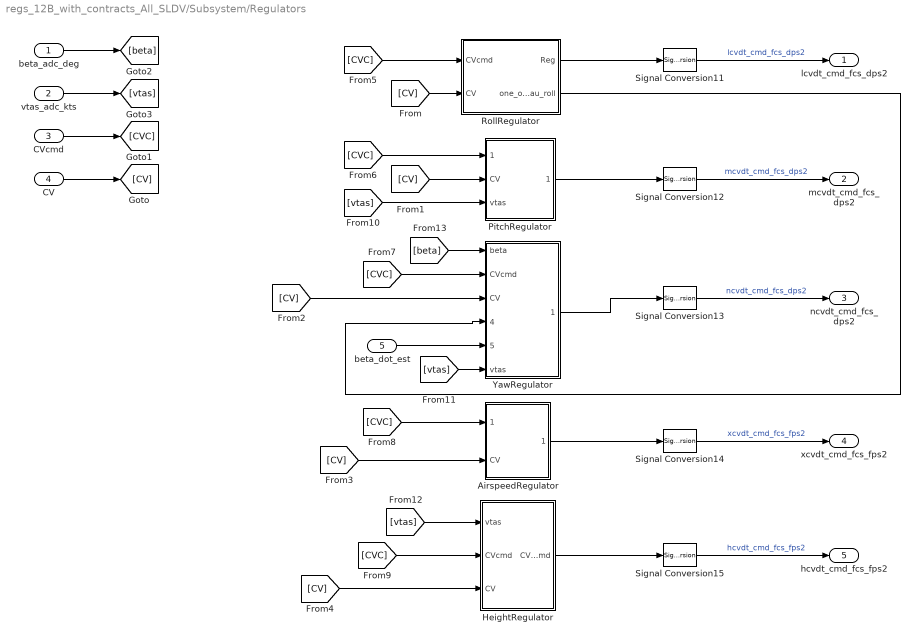
== system regs_12B_with_contracts_All_SLDV/Subsystem/Regulators ==
  beta_adc_deg : Inport
  vtas_adc_kts : Inport  Port=2
  CVcmd : Inport  Port=3
  CV : Inport  Port=4
  beta_dot_est : Inport  Port=5
  AirspeedRegulator : Subsystem
  HeightRegulator : Subsystem
  PitchRegulator : Subsystem
  RollRegulator : Subsystem
  Signal Conversion{11..15} (5 alike) : SignalConversion  ConversionOutput=Contiguous copy  OverrideOpt=on
  YawRegulator : Subsystem
  lcvdt_cmd_fcs_dps2 : Outport  VectorParamsAs1DForOutWhenUnconnected=off
  mcvdt_cmd_fcs_dps2 : Outport  Port=2  VectorParamsAs1DForOutWhenUnconnected=off
  ncvdt_cmd_fcs_dps2 : Outport  Port=3  VectorParamsAs1DForOutWhenUnconnected=off
  xcvdt_cmd_fcs_fps2 : Outport  Port=4  VectorParamsAs1DForOutWhenUnconnected=off
  hcvdt_cmd_fcs_fps2 : Outport  Port=5  VectorParamsAs1DForOutWhenUnconnected=off
  wires:
  RollRegulator/1(Reg) -> Signal Conversion11/1
  PitchRegulator/1(CVdt_cmd) -> Signal Conversion12/1
  YawRegulator/1(CVdt_cmd) -> Signal Conversion13/1
  AirspeedRegulator/1(CVdt_cmd) -> Signal Conversion14/1
  HeightRegulator/1(CVdt_cmd) -> Signal Conversion15/1
  [CVC] -> HeightRegulator/2(CVcmd)
  [CVC] -> YawRegulator/2(CVcmd)
  Signal Conversion11/1 -> lcvdt_cmd_fcs_dps2/1  "lcvdt_cmd_fcs_dps2"
  Signal Conversion12/1 -> mcvdt_cmd_fcs_dps2/1  "mcvdt_cmd_fcs_dps2"
  Signal Conversion13/1 -> ncvdt_cmd_fcs_dps2/1  "ncvdt_cmd_fcs_dps2"
  Signal Conversion15/1 -> hcvdt_cmd_fcs_fps2/1  "hcvdt_cmd_fcs_fps2"
  Signal Conversion14/1 -> xcvdt_cmd_fcs_fps2/1  "xcvdt_cmd_fcs_fps2"
  RollRegulator/2(one_over_Tau_roll) -> YawRegulator/4(one_over_Tau_roll)
  beta_dot_est/1 -> YawRegulator/5(beta_dot_est)
  CV/1 -> [CV]
  [CV] -> RollRegulator/2(CV)
  [CV] -> PitchRegulator/2(CV)
  [CV] -> YawRegulator/3(CV)
  [CV] -> AirspeedRegulator/2(CV)
  [CV] -> HeightRegulator/3(CV)
  CVcmd/1 -> [CVC]
  [CVC] -> RollRegulator/1(CVcmd)
  [CVC] -> PitchRegulator/1(CV_cmd)
  [CVC] -> AirspeedRegulator/1(CVcmd)
  [vtas] -> PitchRegulator/3(vtas)
  [vtas] -> HeightRegulator/1(vtas)
  beta_adc_deg/1 -> [beta]
  vtas_adc_kts/1 -> [vtas]
  [vtas] -> YawRegulator/6(vtas)
  [beta] -> YawRegulator/1(beta)

== system regs_12B_with_contracts_All_SLDV/regs_12B_RegulatorSpec/REG001 ==
  In1 : Inport
  guarantee : Outport  OutDataTypeStr=boolean
  wires:
  In1/1 -> guarantee/1

== system regs_12B_with_contracts_All_SLDV/regs_12B_RegulatorSpec/REG0010 ==
  In1 : Inport
  guarantee : Outport  OutDataTypeStr=boolean
  wires:
  In1/1 -> guarantee/1

== system regs_12B_with_contracts_All_SLDV/regs_12B_RegulatorSpec/REG002 ==
  In1 : Inport
  guarantee : Outport  OutDataTypeStr=boolean
  wires:
  In1/1 -> guarantee/1

== system regs_12B_with_contracts_All_SLDV/regs_12B_RegulatorSpec/REG003 ==
  In1 : Inport
  guarantee : Outport  OutDataTypeStr=boolean
  wires:
  In1/1 -> guarantee/1

== system regs_12B_with_contracts_All_SLDV/regs_12B_RegulatorSpec/REG004 ==
  In1 : Inport
  guarantee : Outport  OutDataTypeStr=boolean
  wires:
  In1/1 -> guarantee/1

== system regs_12B_with_contracts_All_SLDV/regs_12B_RegulatorSpec/REG005 ==
  In1 : Inport
  guarantee : Outport  OutDataTypeStr=boolean
  wires:
  In1/1 -> guarantee/1

== system regs_12B_with_contracts_All_SLDV/regs_12B_RegulatorSpec/REG006 ==
  In1 : Inport
  guarantee : Outport  OutDataTypeStr=boolean
  wires:
  In1/1 -> guarantee/1

== system regs_12B_with_contracts_All_SLDV/regs_12B_RegulatorSpec/REG007 ==
  In1 : Inport
  guarantee : Outport  OutDataTypeStr=boolean
  wires:
  In1/1 -> guarantee/1

== system regs_12B_with_contracts_All_SLDV/regs_12B_RegulatorSpec/REG008 ==
  In1 : Inport
  guarantee : Outport  OutDataTypeStr=boolean
  wires:
  In1/1 -> guarantee/1

== system regs_12B_with_contracts_All_SLDV/regs_12B_RegulatorSpec/REG009 ==
  In1 : Inport
  guarantee : Outport  OutDataTypeStr=boolean
  wires:
  In1/1 -> guarantee/1

== system regs_12B_with_contracts_All_SLDV/Subsystem/Inputs/CVcmd ==
  "lcv_cmd_fcs_dps " : Inport
  hdg_des_deg : Inport  Port=2
  mcv_cmd_fcs_dps : Inport  Port=3
  alt_des_ft : Inport  Port=4
  ncv_cmd_fcs_dps : Inport  Port=5
  xcv_cmd_fcs_fps : Inport  Port=6
  airspeed_des_fps : Inport  Port=7
  hcv_cmd_fcs_fps : Inport  Port=8
  Bus Creator : BusCreator  Inputs=8
  OL_Cmds : Outport  VectorParamsAs1DForOutWhenUnconnected=off
  wires:
  "lcv_cmd_fcs_dps "/1 -> Bus Creator/1  "lcv_cmd_fcs_dps"
  mcv_cmd_fcs_dps/1 -> Bus Creator/3  "mcv_cmd_fcs_dps"
  ncv_cmd_fcs_dps/1 -> Bus Creator/5  "ncv_cmd_fcs_dps"
  xcv_cmd_fcs_fps/1 -> Bus Creator/6  "xcv_cmd_fcs_fps"
  hcv_cmd_fcs_fps/1 -> Bus Creator/8  "hcv_cmd_fcs_fps"
  Bus Creator/1 -> OL_Cmds/1
  hdg_des_deg/1 -> Bus Creator/2  "hdg_des_deg"
  alt_des_ft/1 -> Bus Creator/4  "alt_des_ft"
  airspeed_des_fps/1 -> Bus Creator/7  "airspeed_des_fps"

== system regs_12B_with_contracts_All_SLDV/Subsystem/Inputs/Input ==
  beta_adc_deg : Inport
  vtas_adc_kts : Inport  Port=2
  egi_fcs_in : Subsystem
  beta : Outport  VectorParamsAs1DForOutWhenUnconnected=off
  vtas : Outport  Port=2  VectorParamsAs1DForOutWhenUnconnected=off
  wires:
  beta_adc_deg/1 -> egi_fcs_in/1(beta_adc_deg)  "beta_adc_deg"
  vtas_adc_kts/1 -> egi_fcs_in/2(vtas_adc_kts)  "vtas_adc_kts"
  egi_fcs_in/1(beta_deg) -> beta/1
  egi_fcs_in/2(vtas_kts) -> vtas/1

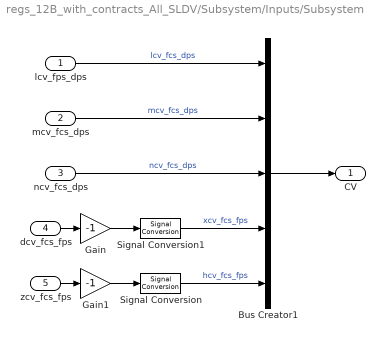
== system regs_12B_with_contracts_All_SLDV/Subsystem/Inputs/Subsystem ==
  lcv_fps_dps : Inport
  mcv_fcs_dps : Inport  Port=2
  ncv_fcs_dps : Inport  Port=3
  dcv_fcs_fps : Inport  Port=4
  zcv_fcs_fps : Inport  Port=5
  Bus Creator1 : BusCreator  Inputs=5
  Gain : Gain  Gain=-1
  Gain1 : Gain  Gain=-1
  Signal Conversion : SignalConversion  ConversionOutput=Contiguous copy  OverrideOpt=off
  Signal Conversion1 : SignalConversion  ConversionOutput=Contiguous copy  OverrideOpt=off
  CV : Outport  VectorParamsAs1DForOutWhenUnconnected=off
  wires:
  Gain1/1 -> Signal Conversion/1
  zcv_fcs_fps/1 -> Gain1/1
  Signal Conversion1/1 -> Bus Creator1/4  "xcv_fcs_fps"
  Gain/1 -> Signal Conversion1/1
  Bus Creator1/1 -> CV/1
  mcv_fcs_dps/1 -> Bus Creator1/2  "mcv_fcs_dps"
  lcv_fps_dps/1 -> Bus Creator1/1  "lcv_fcs_dps"
  Signal Conversion/1 -> Bus Creator1/5  "hcv_fcs_fps"
  ncv_fcs_dps/1 -> Bus Creator1/3  "ncv_fcs_dps"
  dcv_fcs_fps/1 -> Gain/1

== system regs_12B_with_contracts_All_SLDV/Subsystem/Inputs/betad ==
  betadot : Inport
  beta_dot_est : Outport  VectorParamsAs1DForOutWhenUnconnected=off
  wires:
  betadot/1 -> beta_dot_est/1

== system regs_12B_with_contracts_All_SLDV/Subsystem/Regulators/AirspeedRegulator ==
  note: Speed Regulator
  note: 1 / Tau
  CVcmd : Inport
  CV : Inport  Port=2
  Bus Selector1 : BusSelector  OutputSignals=xcv_cmd_fcs_fps
  Bus Selector2 : BusSelector  OutputSignals=xcv_fcs_fps
  Gain : Gain  Gain=0.5
  Signal Conversion1 : SignalConversion  ConversionOutput=Contiguous copy  OverrideOpt=on
  Signal Conversion12 : SignalConversion  ConversionOutput=Contiguous copy  OverrideOpt=on
  Sum1 : Sum  Inputs=+-|  SaturateOnIntegerOverflow=on  InputSameDT=on  OutDataTypeStr=Inherit: Same as first input
  CVdt_cmd : Outport  VectorParamsAs1DForOutWhenUnconnected=off
  wires:
  Gain/1 -> CVdt_cmd/1  "CVdt_cmd"
  CVcmd/1 -> Bus Selector1/1
  Signal Conversion12/1 -> Sum1/1  "CV_cmd"
  Signal Conversion1/1 -> Sum1/2  "CV"
  CV/1 -> Bus Selector2/1
  Bus Selector2/1 -> Signal Conversion1/1  "<xcv_fcs_fps>"
  Bus Selector1/1 -> Signal Conversion12/1  "<xcv_cmd_fcs_fps>"
  Sum1/1 -> Gain/1  "CV_err"

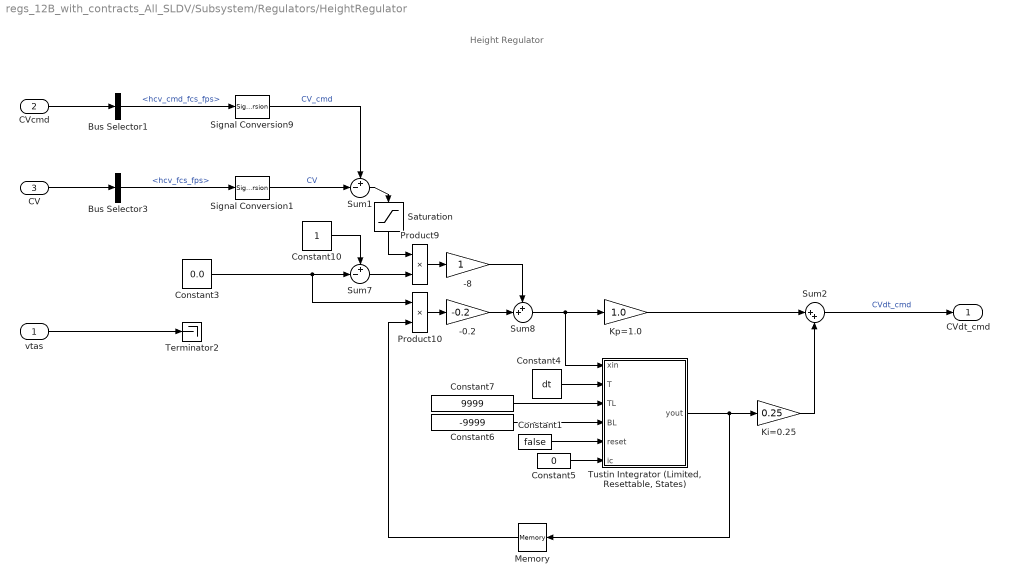
== system regs_12B_with_contracts_All_SLDV/Subsystem/Regulators/HeightRegulator ==
  note: Height Regulator
  vtas : Inport
  CVcmd : Inport  Port=2
  CV : Inport  Port=3
  -0.2 : Gain  Gain=-0.2
  -8 : Gain
  Bus Selector1 : BusSelector  OutputSignals=hcv_cmd_fcs_fps
  Bus Selector3 : BusSelector  OutputSignals=hcv_fcs_fps
  Constant1 : Constant  Value=false
  Constant10 : Constant
  Constant3 : Constant  Value=0.0
  Constant4 : Constant  Value=dt
  Constant5 : Constant  Value=0
  Constant6 : Constant  Value=-9999
  Constant7 : Constant  Value=9999
  Ki=0.25 : Gain  Gain=0.25
  Kp=1.0 : Gain  Gain=1.0
  Memory : Memory
  Product10 : Product  SaturateOnIntegerOverflow=on  OutDataTypeStr=Inherit: Same as first input
  Product9 : Product  SaturateOnIntegerOverflow=on  OutDataTypeStr=Inherit: Same as first input
  Saturation : Saturate  UpperLimit=1  LowerLimit=-1
  Signal Conversion1 : SignalConversion  ConversionOutput=Contiguous copy  OverrideOpt=on
  Signal Conversion9 : SignalConversion  ConversionOutput=Contiguous copy  OverrideOpt=on
  Sum1 : Sum  Inputs=+-|  SaturateOnIntegerOverflow=on  InputSameDT=on  OutDataTypeStr=Inherit: Same as first input
  Sum2 : Sum  Inputs=|++  SaturateOnIntegerOverflow=on  InputSameDT=on  OutDataTypeStr=Inherit: Same as first input
  Sum7 : Sum  Inputs=+-|
  Sum8 : Sum  Inputs=++|
  Terminator2 : Terminator
  "Tustin Integrator (Limited, Resettable, States)" : Subsystem
  CVdt_cmd : Outport  VectorParamsAs1DForOutWhenUnconnected=off
  wires:
  Bus Selector1/1 -> Signal Conversion9/1  "<hcv_cmd_fcs_fps>"
  CVcmd/1 -> Bus Selector1/1
  Signal Conversion9/1 -> Sum1/1  "CV_cmd"
  Signal Conversion1/1 -> Sum1/2  "CV"
  CV/1 -> Bus Selector3/1
  Bus Selector3/1 -> Signal Conversion1/1  "<hcv_fcs_fps>"
  Sum1/1 -> Saturation/1
  Sum2/1 -> CVdt_cmd/1  "CVdt_cmd"
  Ki=0.25/1 -> Sum2/2
  Kp=1.0/1 -> Sum2/1
  Product9/1 -> -8/1
  Product10/1 -> -0.2/1
  -0.2/1 -> Sum8/2
  -8/1 -> Sum8/1
  Sum7/1 -> Product9/2
  Constant3/1 -> Sum7/2, Product10/1
  Constant10/1 -> Sum7/1
  Sum8/1 -> "Tustin Integrator (Limited, Resettable, States)"/1(xin), Kp=1.0/1
  Memory/1 -> Product10/2
  vtas/1 -> Terminator2/1
  Saturation/1 -> Product9/1
  Constant4/1 -> "Tustin Integrator (Limited, Resettable, States)"/2(T)
  Constant7/1 -> "Tustin Integrator (Limited, Resettable, States)"/3(TL)
  Constant6/1 -> "Tustin Integrator (Limited, Resettable, States)"/4(BL)
  Constant1/1 -> "Tustin Integrator (Limited, Resettable, States)"/5(reset)
  Constant5/1 -> "Tustin Integrator (Limited, Resettable, States)"/6(ic)
  "Tustin Integrator (Limited, Resettable, States)"/1(yout) -> Memory/1, Ki=0.25/1

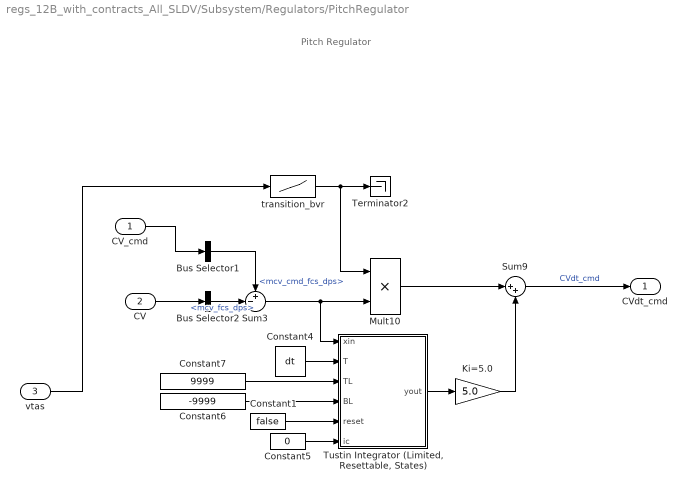
== system regs_12B_with_contracts_All_SLDV/Subsystem/Regulators/PitchRegulator ==
  note: Pitch Regulator
  CV_cmd : Inport
  CV : Inport  Port=2
  vtas : Inport  Port=3
  Bus Selector1 : BusSelector  OutputSignals=mcv_cmd_fcs_dps
  Bus Selector2 : BusSelector  OutputSignals=mcv_fcs_dps
  Constant1 : Constant  Value=false
  Constant4 : Constant  Value=dt
  Constant5 : Constant  Value=0
  Constant6 : Constant  Value=-9999
  Constant7 : Constant  Value=9999
  Ki=5.0 : Gain  Gain=5.0
  Mult10 : Product  SaturateOnIntegerOverflow=on  InputSameDT=on  OutDataTypeStr=Inherit: Same as first input
  Sum3 : Sum  Inputs=+-|  SaturateOnIntegerOverflow=on  InputSameDT=on  OutDataTypeStr=Inherit: Same as first input
  Sum9 : Sum  Inputs=|++  SaturateOnIntegerOverflow=on  InputSameDT=on  OutDataTypeStr=Inherit: Same as first input
  Terminator2 : Terminator
  "Tustin Integrator (Limited, Resettable, States)" : Subsystem
  transition_bvr : Lookup_n-D  NumberOfTableDimensions=1  BreakpointsForDimension1=[120 185]  Table=[15 20]  InternalRulePriority=Speed  InputSameDT=on
  CVdt_cmd : Outport  VectorParamsAs1DForOutWhenUnconnected=off
  wires:
  CV_cmd/1 -> Bus Selector1/1
  CV/1 -> Bus Selector2/1
  Constant4/1 -> "Tustin Integrator (Limited, Resettable, States)"/2(T)
  Constant5/1 -> "Tustin Integrator (Limited, Resettable, States)"/6(ic)
  "Tustin Integrator (Limited, Resettable, States)"/1(yout) -> Ki=5.0/1
  Mult10/1 -> Sum9/1
  Ki=5.0/1 -> Sum9/2
  Sum9/1 -> CVdt_cmd/1  "CVdt_cmd"
  Bus Selector1/1 -> Sum3/1  "<mcv_cmd_fcs_dps>"
  Bus Selector2/1 -> Sum3/2  "<mcv_fcs_dps>"
  transition_bvr/1 -> Terminator2/1, Mult10/1
  Constant1/1 -> "Tustin Integrator (Limited, Resettable, States)"/5(reset)
  vtas/1 -> transition_bvr/1
  Sum3/1 -> "Tustin Integrator (Limited, Resettable, States)"/1(xin), Mult10/2
  Constant6/1 -> "Tustin Integrator (Limited, Resettable, States)"/4(BL)
  Constant7/1 -> "Tustin Integrator (Limited, Resettable, States)"/3(TL)

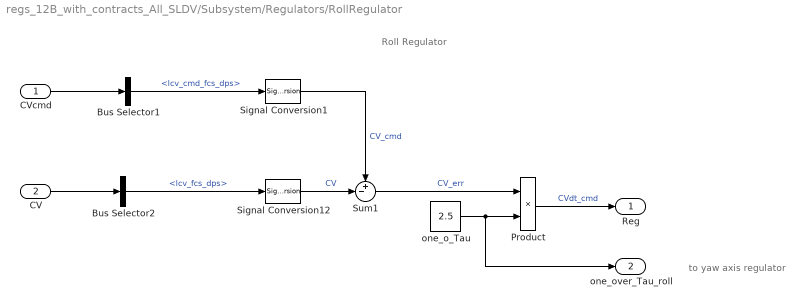
== system regs_12B_with_contracts_All_SLDV/Subsystem/Regulators/RollRegulator ==
  note: Roll Regulator
  note: to yaw axis regulator
  CVcmd : Inport
  CV : Inport  Port=2
  Bus Selector1 : BusSelector  OutputSignals=lcv_cmd_fcs_dps
  Bus Selector2 : BusSelector  OutputSignals=lcv_fcs_dps
  Product : Product  RndMeth=Zero
  Signal Conversion1 : SignalConversion  ConversionOutput=Contiguous copy  OverrideOpt=on
  Signal Conversion12 : SignalConversion  ConversionOutput=Contiguous copy  OverrideOpt=on
  Sum1 : Sum  Inputs=+-|  SaturateOnIntegerOverflow=on  InputSameDT=on  OutDataTypeStr=Inherit: Same as first input
  one_o_Tau : Constant  Value=2.5
  Reg : Outport  VectorParamsAs1DForOutWhenUnconnected=off
  one_over_Tau_roll : Outport  Port=2  VectorParamsAs1DForOutWhenUnconnected=off
  wires:
  Sum1/1 -> Product/1  "CV_err"
  Signal Conversion1/1 -> Sum1/1  "CV_cmd"
  Signal Conversion12/1 -> Sum1/2  "CV"
  CV/1 -> Bus Selector2/1
  Bus Selector2/1 -> Signal Conversion12/1  "<lcv_fcs_dps>"
  Bus Selector1/1 -> Signal Conversion1/1  "<lcv_cmd_fcs_dps>"
  CVcmd/1 -> Bus Selector1/1
  one_o_Tau/1 -> Product/2, one_over_Tau_roll/1
  Product/1 -> Reg/1  "CVdt_cmd"

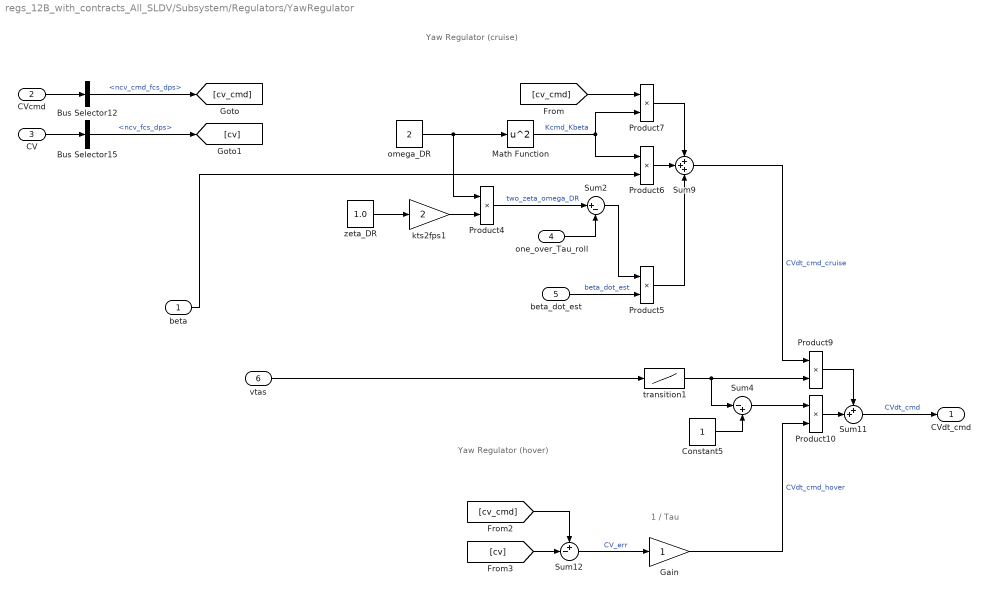
== system regs_12B_with_contracts_All_SLDV/Subsystem/Regulators/YawRegulator ==
  note: Yaw Regulator (hover)
  note: 1 / Tau
  note: Yaw Regulator (cruise)
  beta : Inport
  CVcmd : Inport  Port=2
  CV : Inport  Port=3
  one_over_Tau_roll : Inport  Port=4
  beta_dot_est : Inport  Port=5
  vtas : Inport  Port=6
  Bus Selector12 : BusSelector  OutputSignals=ncv_cmd_fcs_dps
  Bus Selector15 : BusSelector  OutputSignals=ncv_fcs_dps
  Constant5 : Constant
  Gain : Gain
  Math Function : Math  Operator=square  SaturateOnIntegerOverflow=on
  Product{4..7,9..10} (6 alike) : Product  SaturateOnIntegerOverflow=on  OutDataTypeStr=Inherit: Same as first input
  Sum11 : Sum  Inputs=++|
  Sum12 : Sum  Inputs=+-|  SaturateOnIntegerOverflow=on  InputSameDT=on  OutDataTypeStr=Inherit: Same as first input
  Sum2 : Sum  Inputs=|+-  SaturateOnIntegerOverflow=on  InputSameDT=on  OutDataTypeStr=Inherit: Same as first input
  Sum4 : Sum  Inputs=|-+
  Sum9 : Sum  Inputs=+++  SaturateOnIntegerOverflow=on  InputSameDT=on  OutDataTypeStr=Inherit: Same as first input
  kts2fps1 : Gain  Gain=2
  omega_DR : Constant  Value=2
  transition1 : Lookup_n-D  NumberOfTableDimensions=1  BreakpointsForDimension1=transition_v  Table=transition_y  InternalRulePriority=Speed  InputSameDT=on
  zeta_DR : Constant  Value=1.0
  CVdt_cmd : Outport  VectorParamsAs1DForOutWhenUnconnected=off
  wires:
  beta/1 -> Product6/2
  Product6/1 -> Sum9/2
  omega_DR/1 -> Math Function/1, Product4/1
  Product7/1 -> Sum9/1
  Math Function/1 -> Product6/1, Product7/2  "Kcmd_Kbeta"
  Sum11/1 -> CVdt_cmd/1  "CVdt_cmd"
  transition1/1 -> Sum4/1, Product9/2
  Product9/1 -> Sum11/1
  Constant5/1 -> Sum4/2
  Sum4/1 -> Product10/1
  Product10/1 -> Sum11/2
  Sum9/1 -> Product9/1  "CVdt_cmd_cruise"
  Sum12/1 -> Gain/1  "CV_err"
  Bus Selector12/1 -> [cv_cmd]  "<ncv_cmd_fcs_dps>"
  CVcmd/1 -> Bus Selector12/1
  CV/1 -> Bus Selector15/1
  Bus Selector15/1 -> [cv]  "<ncv_fcs_dps>"
  beta_dot_est/1 -> Product5/2  "beta_dot_est"
  Gain/1 -> Product10/2  "CVdt_cmd_hover"
  [cv_cmd] -> Product7/1
  [cv_cmd] -> Sum12/1
  [cv] -> Sum12/2
  zeta_DR/1 -> kts2fps1/1
  kts2fps1/1 -> Product4/2
  Product4/1 -> Sum2/1  "two_zeta_omega_DR"
  one_over_Tau_roll/1 -> Sum2/2
  Product5/1 -> Sum9/3
  Sum2/1 -> Product5/1
  vtas/1 -> transition1/1

== system regs_12B_with_contracts_All_SLDV/Subsystem/Inputs/Input/egi_fcs_in ==
  beta_adc_deg : Inport
  vtas_adc_kts : Inport  Port=2
  beta_deg : Outport  VectorParamsAs1DForOutWhenUnconnected=off
  vtas_kts : Outport  Port=2  VectorParamsAs1DForOutWhenUnconnected=off
  wires:
  beta_adc_deg/1 -> beta_deg/1  "beta_adc_deg"
  vtas_adc_kts/1 -> vtas_kts/1  "vtas_adc_kts"

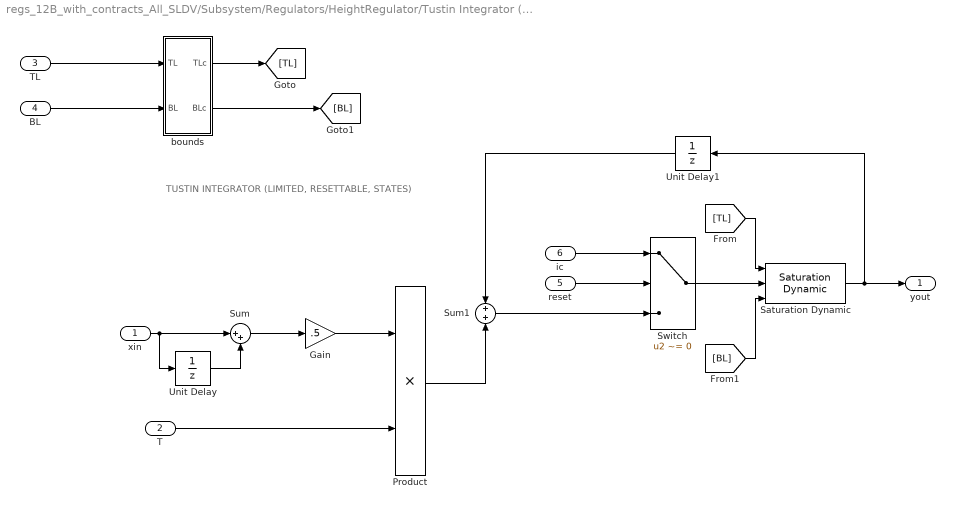
== system regs_12B_with_contracts_All_SLDV/Subsystem/Regulators/HeightRegulator/Tustin Integrator (Limited, Resettable, States) ==
  note: TUSTIN INTEGRATOR (LIMITED, RESETTABLE, STATES)
  xin : Inport
  T : Inport  Port=2
  TL : Inport  Port=3
  BL : Inport  Port=4
  reset : Inport  Port=5
  ic : Inport  Port=6
  Gain : Gain  Gain=.5
  Product : Product  RndMeth=Zero
  Saturation Dynamic : simulink/Discontinuities/Saturation Dynamic  OutMin=[]  OutMax=[]  OutDataTypeStr=Inherit: Same as second input  OutDataType=fixdt(1, 16)  OutScaling=2^-10  DoSatur=off
  Sum : Sum  Inputs=|++
  Sum1 : Sum
  Switch : Switch  Criteria=u2 ~= 0  Threshold=0.5
  Unit Delay : UnitDelay  SampleTime=-1  HasFrameUpgradeWarning=on
  Unit Delay1 : UnitDelay  SampleTime=-1  HasFrameUpgradeWarning=on
  bounds : Subsystem
  yout : Outport  VectorParamsAs1DForOutWhenUnconnected=off
  wires:
  xin/1 -> Unit Delay/1, Sum/1
  Unit Delay/1 -> Sum/2
  Sum/1 -> Gain/1
  Gain/1 -> Product/1
  T/1 -> Product/2
  Product/1 -> Sum1/2
  Sum1/1 -> Switch/3
  reset/1 -> Switch/2
  ic/1 -> Switch/1
  Switch/1 -> Saturation Dynamic/2
  Saturation Dynamic/1 -> Unit Delay1/1, yout/1
  Unit Delay1/1 -> Sum1/1
  TL/1 -> bounds/1(TL)
  BL/1 -> bounds/2(BL)
  bounds/1(TLc) -> [TL]
  bounds/2(BLc) -> [BL]
  [TL] -> Saturation Dynamic/1
  [BL] -> Saturation Dynamic/3

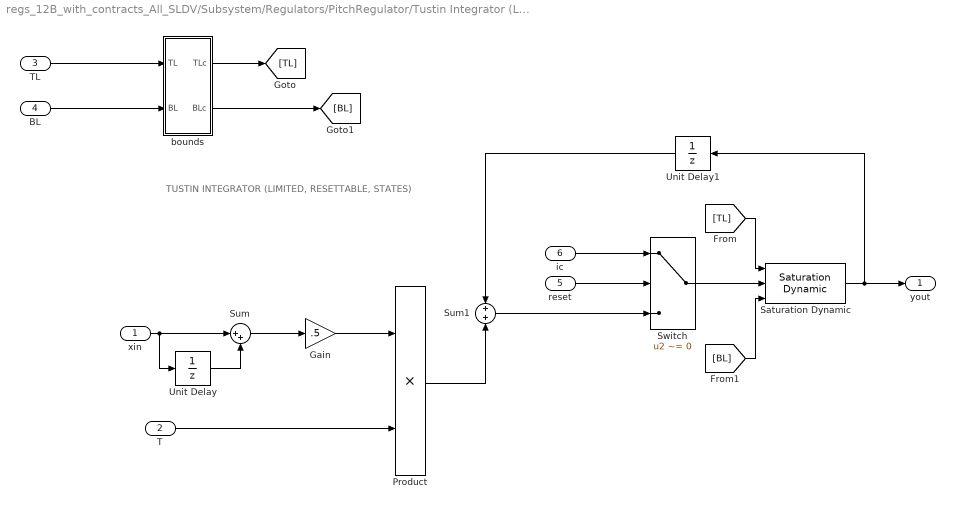
== system regs_12B_with_contracts_All_SLDV/Subsystem/Regulators/PitchRegulator/Tustin Integrator (Limited, Resettable, States) ==
  note: TUSTIN INTEGRATOR (LIMITED, RESETTABLE, STATES)
  xin : Inport
  T : Inport  Port=2
  TL : Inport  Port=3
  BL : Inport  Port=4
  reset : Inport  Port=5
  ic : Inport  Port=6
  Gain : Gain  Gain=.5
  Product : Product  RndMeth=Zero
  Saturation Dynamic : simulink/Discontinuities/Saturation Dynamic  OutMin=[]  OutMax=[]  OutDataTypeStr=Inherit: Same as second input  OutDataType=fixdt(1, 16)  OutScaling=2^-10  DoSatur=off
  Sum : Sum  Inputs=|++
  Sum1 : Sum
  Switch : Switch  Criteria=u2 ~= 0  Threshold=0.5
  Unit Delay : UnitDelay  SampleTime=-1  HasFrameUpgradeWarning=on
  Unit Delay1 : UnitDelay  SampleTime=-1  HasFrameUpgradeWarning=on
  bounds : Subsystem
  yout : Outport  VectorParamsAs1DForOutWhenUnconnected=off
  wires:
  xin/1 -> Unit Delay/1, Sum/1
  Unit Delay/1 -> Sum/2
  Sum/1 -> Gain/1
  Gain/1 -> Product/1
  T/1 -> Product/2
  Product/1 -> Sum1/2
  Sum1/1 -> Switch/3
  reset/1 -> Switch/2
  ic/1 -> Switch/1
  Switch/1 -> Saturation Dynamic/2
  Saturation Dynamic/1 -> Unit Delay1/1, yout/1
  Unit Delay1/1 -> Sum1/1
  TL/1 -> bounds/1(TL)
  BL/1 -> bounds/2(BL)
  bounds/1(TLc) -> [TL]
  bounds/2(BLc) -> [BL]
  [TL] -> Saturation Dynamic/1
  [BL] -> Saturation Dynamic/3

== system regs_12B_with_contracts_All_SLDV/Subsystem/Regulators/HeightRegulator/Tustin Integrator (Limited, Resettable, States)/bounds ==
  TL : Inport
  BL : Inport  Port=2
  Relational Operator : RelationalOperator  Operator=<  OutDataTypeStr=boolean  RndMeth=Nearest
  Switch1 : Switch  Criteria=u2 ~= 0  Threshold=0.5
  Switch2 : Switch  Criteria=u2 ~= 0  Threshold=0.5
  TLc : Outport  VectorParamsAs1DForOutWhenUnconnected=off
  BLc : Outport  Port=2  VectorParamsAs1DForOutWhenUnconnected=off
  wires:
  BL/1 -> Switch1/1, Switch2/3, Relational Operator/2
  TL/1 -> Switch2/1, Switch1/3, Relational Operator/1
  Relational Operator/1 -> Switch2/2, Switch1/2
  Switch1/1 -> TLc/1
  Switch2/1 -> BLc/1

== system regs_12B_with_contracts_All_SLDV/Subsystem/Regulators/PitchRegulator/Tustin Integrator (Limited, Resettable, States)/bounds ==
  TL : Inport
  BL : Inport  Port=2
  Relational Operator : RelationalOperator  Operator=<  OutDataTypeStr=boolean  RndMeth=Nearest
  Switch1 : Switch  Criteria=u2 ~= 0  Threshold=0.5
  Switch2 : Switch  Criteria=u2 ~= 0  Threshold=0.5
  TLc : Outport  VectorParamsAs1DForOutWhenUnconnected=off
  BLc : Outport  Port=2  VectorParamsAs1DForOutWhenUnconnected=off
  wires:
  BL/1 -> Switch1/1, Switch2/3, Relational Operator/2
  TL/1 -> Switch2/1, Switch1/3, Relational Operator/1
  Relational Operator/1 -> Switch2/2, Switch1/2
  Switch1/1 -> TLc/1
  Switch2/1 -> BLc/1
